simulink subsystem "PowerControlSubsystem"  (R2023b)
settings: Solver=VariableStepAuto  StartTime=0.0  StopTime=10.0  RelTol=1e-3
values from neighbouring files (symbols this model uses):
  controllerTimeConstant = 2    [wind_turbine_inputs.m]
  generatorEfficiency = 90    [wind_turbine_inputs.m]
  pGeneratorBrakeLimit = 0.50    (= 0.5)    [wind_turbine_inputs.m]
  turbineRatedPower = 1.5    [wind_turbine_inputs.m]
  vWindRated = 12    [wind_turbine_inputs.m]
  wAtGeneratorRatedPower = wTurbineCutOut*gearRatio    (= 1227.93)    [wind_turbine_inputs.m]
  wGeneratorBrakeLimit = 0.50    (= 0.5)    [wind_turbine_inputs.m]
undefined symbols (not defined in the file or in its folder): mpptOmega, mpptPower, mpptWindSpeed
libraries: simulink x2
settings Model: Creator=FRESH  LastModifiedBy=FRESH

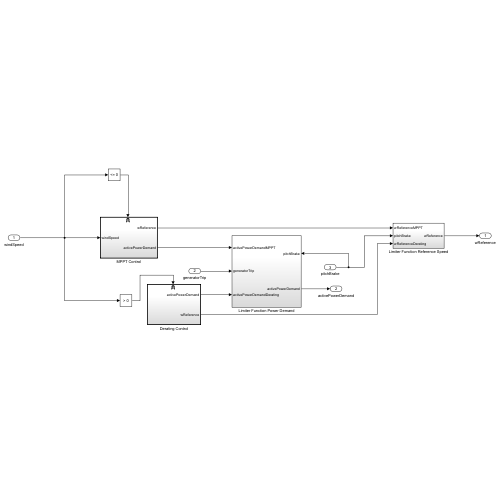
[thumbnail: Simulink's stored preview of the top-level diagram]
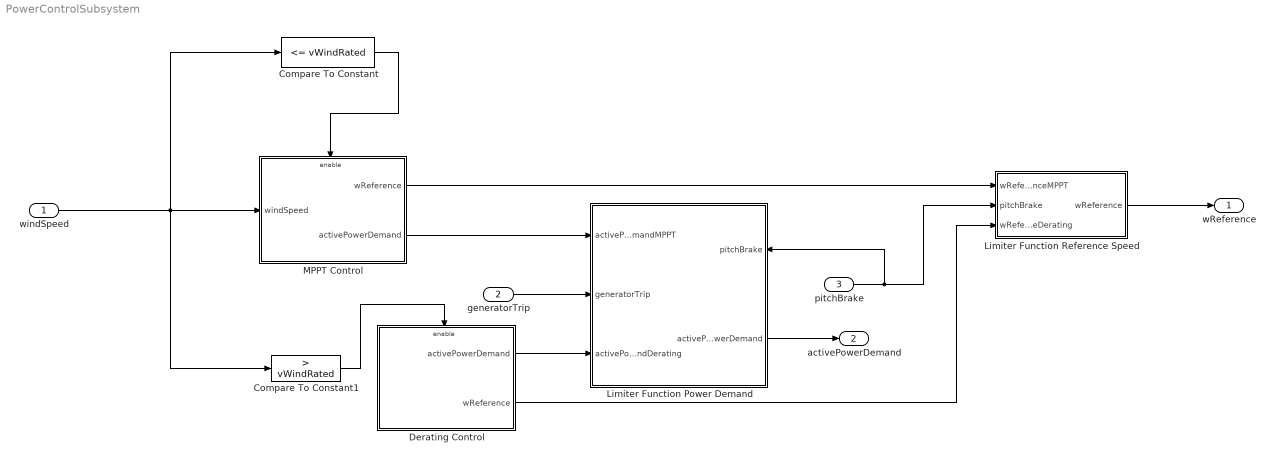
== system PowerControlSubsystem ==
  windSpeed : Inport
  generatorTrip : Inport  Port=2
  pitchBrake : Inport  Port=3
  Compare To Constant : simulink/Logic and Bit Operations/Compare To Constant  relop=<=  const=vWindRated  OutDataTypeStr=boolean
  Compare To Constant1 : simulink/Logic and Bit Operations/Compare To Constant  relop=>  const=vWindRated  OutDataTypeStr=boolean
  Derating Control : Subsystem
  Limiter Function Power Demand : Subsystem
      settings: PortSchema="{\"entries\":[{\"content\":{\"sides\":[{\"content\":{\"connectorIds\":[\"In1\",\"In2\",\"In3\"]},\"type\":\"ConnectorPlacement.EquallySpacedRectSide\",\"uuid\":\"b03cf57d-370b-4fa1-bd93-9b836e03697e\"},{\"content\":{\"connectorIds\":[\"In4\",\"Out1\"],\"side\":\"RIGHT\"},\"type\":\"ConnectorPlacement.EquallySpacedRectSide\",\"uuid\":\"152758c3-43df-447a-a50f-afca466b3eeb\"},{\"content\":{\"connectorIds\":[],\"side\":\"TOP\"},\"type\":\"ConnectorPlacement.EquallySpacedRectSide\",\"uuid\":\"d053be3f-8f1f-4fa1-8d53-3d41a1fdecc7\"}]},\"type\":\"ConnectorPlacement.EquallySpacedConnector\",\"uuid\":\"ad588a80-a06e-49b6-a4d2-a4be271ff49a\"}],\"packageUris\":[\"http://schema.mathworks.com/mf0/Connector/R2020b\"],\"version\":\"1.0\"}"
  Limiter Function Reference Speed : Subsystem
  MPPT Control : Subsystem
  wReference : Outport
  activePowerDemand : Outport  Port=2
  wires:
  Compare To Constant/1 -> MPPT Control/Enable
  windSpeed/1 -> Compare To Constant1/1, Compare To Constant/1, MPPT Control/1(windSpeed)
  Compare To Constant1/1 -> Derating Control/Enable
  MPPT Control/2(activePowerDemand) -> Limiter Function Power Demand/1(activePowerDemandMPPT)
  MPPT Control/1(wReference) -> Limiter Function Reference Speed/1(wReferenceMPPT)
  Limiter Function Reference Speed/1(wReference) -> wReference/1
  generatorTrip/1 -> Limiter Function Power Demand/2(generatorTrip)
  Limiter Function Power Demand/1(activePowerDemand) -> activePowerDemand/1
  pitchBrake/1 -> Limiter Function Power Demand/4(pitchBrake), Limiter Function Reference Speed/2(pitchBrake)
  Derating Control/1(activePowerDemand) -> Limiter Function Power Demand/3(activePowerDemandDerating)
  Derating Control/2(wReference) -> Limiter Function Reference Speed/3(wReferenceDerating)

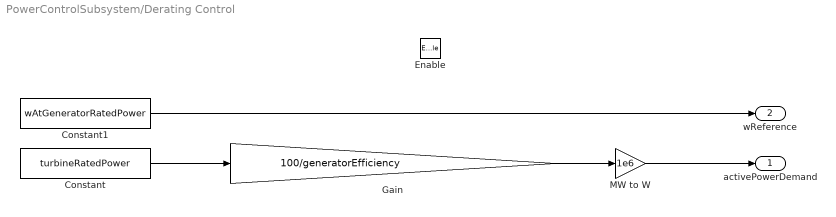
== system PowerControlSubsystem/Derating Control ==
  Enable : EnablePort  StatesWhenEnabling=reset
  Constant : Constant  Value=turbineRatedPower
  Constant1 : Constant  Value=wAtGeneratorRatedPower
  Gain : Gain  Gain=100/generatorEfficiency
  MW to W : Gain  Gain=1e6
  activePowerDemand : Outport
  wReference : Outport  Port=2
  wires:
  Constant1/1 -> wReference/1
  MW to W/1 -> activePowerDemand/1
  Constant/1 -> Gain/1
  Gain/1 -> MW to W/1

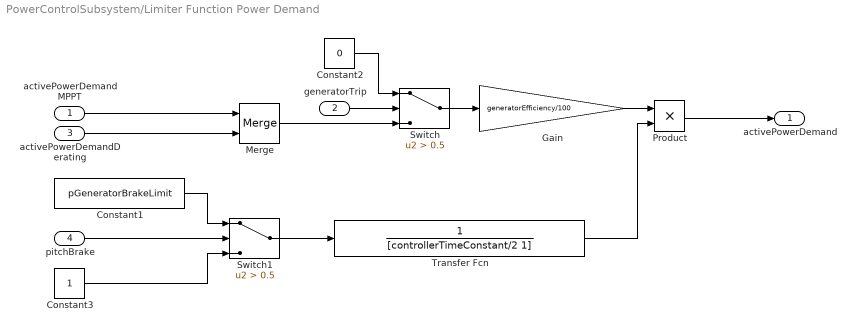
== system PowerControlSubsystem/Limiter Function Power Demand ==
  activePowerDemandMPPT : Inport
  generatorTrip : Inport  Port=2
  activePowerDemandDerating : Inport  Port=3
  pitchBrake : Inport  Port=4
  Constant1 : Constant  Value=pGeneratorBrakeLimit
  Constant2 : Constant  Value=0
  Constant3 : Constant
  Gain : Gain  Gain=generatorEfficiency/100
  Merge : Merge
  Product : Product
  Switch : Switch  Criteria=u2 > Threshold  Threshold=0.5  SaturateOnIntegerOverflow=off  InputSameDT=off
  Switch1 : Switch  Criteria=u2 > Threshold  Threshold=0.5  SaturateOnIntegerOverflow=off  InputSameDT=off
  Transfer Fcn : TransferFcn  Denominator=[controllerTimeConstant/2 1]
  activePowerDemand : Outport
  wires:
  generatorTrip/1 -> Switch/2
  Switch/1 -> Gain/1
  Constant2/1 -> Switch/1
  Merge/1 -> Switch/3
  activePowerDemandMPPT/1 -> Merge/1
  activePowerDemandDerating/1 -> Merge/2
  pitchBrake/1 -> Switch1/2
  Constant3/1 -> Switch1/3
  Constant1/1 -> Switch1/1
  Gain/1 -> Product/1
  Switch1/1 -> Transfer Fcn/1
  Product/1 -> activePowerDemand/1
  Transfer Fcn/1 -> Product/2

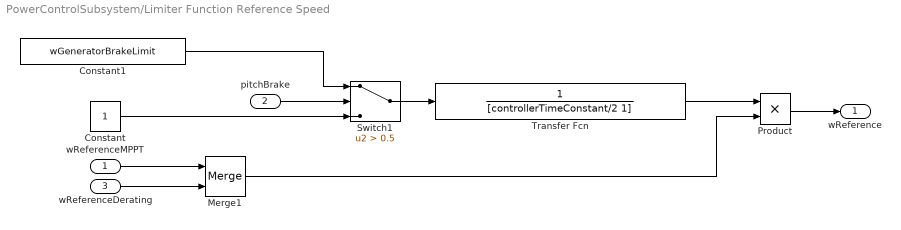
== system PowerControlSubsystem/Limiter Function Reference Speed ==
  wReferenceMPPT : Inport
  pitchBrake : Inport  Port=2
  wReferenceDerating : Inport  Port=3
  Constant : Constant
  Constant1 : Constant  Value=wGeneratorBrakeLimit
  Merge1 : Merge
  Product : Product
  Switch1 : Switch  Criteria=u2 > Threshold  Threshold=0.5  SaturateOnIntegerOverflow=off  InputSameDT=off
  Transfer Fcn : TransferFcn  Denominator=[controllerTimeConstant/2 1]
  wReference : Outport
  wires:
  pitchBrake/1 -> Switch1/2
  Constant1/1 -> Switch1/1
  wReferenceMPPT/1 -> Merge1/1
  wReferenceDerating/1 -> Merge1/2
  Merge1/1 -> Product/2
  Constant/1 -> Switch1/3
  Product/1 -> wReference/1
  Transfer Fcn/1 -> Product/1
  Switch1/1 -> Transfer Fcn/1

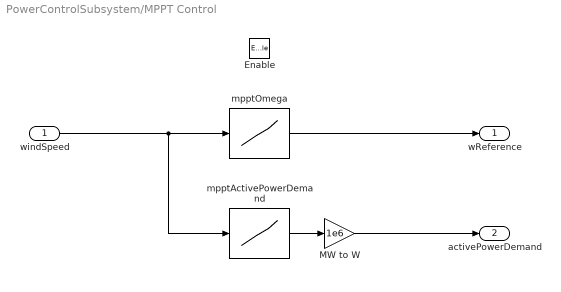
== system PowerControlSubsystem/MPPT Control ==
  windSpeed : Inport
  Enable : EnablePort  StatesWhenEnabling=reset
  MW to W : Gain  Gain=1e6
  mpptActivePowerDemand : Lookup_n-D  NumberOfTableDimensions=1  BreakpointsForDimension1=mpptWindSpeed  Table=mpptPower  InternalRulePriority=Speed  RndMeth=Simplest
  mpptOmega : Lookup_n-D  NumberOfTableDimensions=1  BreakpointsForDimension1=mpptWindSpeed  Table=mpptOmega  InternalRulePriority=Speed  RndMeth=Simplest
  wReference : Outport
  activePowerDemand : Outport  Port=2
  wires:
  mpptActivePowerDemand/1 -> MW to W/1
  mpptOmega/1 -> wReference/1
  windSpeed/1 -> mpptActivePowerDemand/1, mpptOmega/1
  MW to W/1 -> activePowerDemand/1
